simulink model "Lab_3_BD1_Reduce"  (R2024a)
settings: Solver=VariableStepAuto  StartTime=0.0  StopTime=20  RelTol=1e-3
values from neighbouring files (symbols this model uses):
  G4_den = [1 -1 0 0 1 -2 1]    [Lab_3_BD1.m]    (also in Laboratory_3_No_2.m = [2 0])
  G4_num = [1 0 -4 0]    [Lab_3_BD1.m]    (also in Laboratory_3_No_2.m = [1])
settings Model: LastModifiedBy=Sydney Ruoj

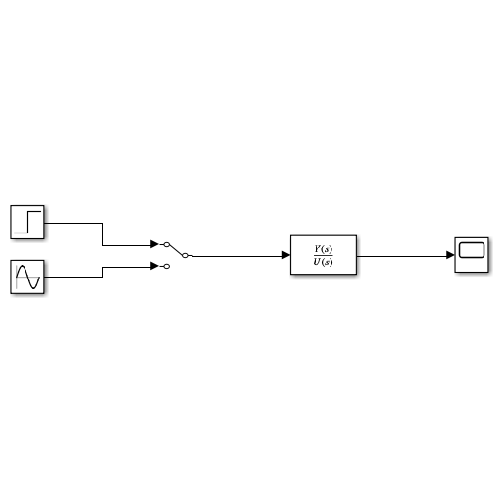
[thumbnail: Simulink's stored preview of the top-level diagram]
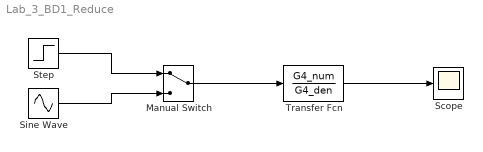
== system Lab_3_BD1_Reduce ==
  Manual Switch : ManualSwitch
  Scope : Scope
  Sine Wave : Sin  SampleTime=0
  Step : Step  Time=0  SampleTime=0
  Transfer Fcn : TransferFcn  Numerator=G4_num  Denominator=G4_den
  wires:
  Sine Wave/1 -> Manual Switch/2
  Transfer Fcn/1 -> Scope/1
  Manual Switch/1 -> Transfer Fcn/1
  Step/1 -> Manual Switch/1
